simulink model "sgMdl_IO3xx_SPI_Loopback_MasterSyncMultiSlave"  (R2024b)
settings: Solver=FixedStepAuto  StartTime=0.0  StopTime=inf  RelTol=1e-3  EnableMultiTasking=on
undefined symbols (not defined in the file): Pull, pull, up
libraries: simulink x2, speedgoatlib_fpga_spi x2, speedgoatlib_fpga x1
Description:
  | IO3xx SPI - Loopback Master Sync MultiSlave
settings Model: ModifiedByFormat=Speedgoat  SimulationMode=external  ExtModeTrigDuration=100000  Creator=Speedgoat  LastModifiedBy=Speedgoat
settings SolverCC: ConcurrentTasks=on  AlgebraicLoopSolver=TrustRegion  PositivePriorityOrder=on  InsertRTBMode=Never (minimum delay)
settings DataIOCC: SaveFormat=Array  SaveState=on  SignalLoggingName=logsOut
settings OptimizationCC: BlockReduction=off  BooleanDataType=off  OptimizeBlockIOStorage=off  BufferReuse=off  ReuseModelBlockBuffer=off  GlobalBufferReuse=off  ExpressionFolding=off  LocalBlockOutputs=off  InitFltsAndDblsToZero=on  OptimizeDataStoreBuffers=off  BusAssignmentInplaceUpdate=off
settings DebuggingCC: SaveWithParameterizedLinksMsg=none  UnderspecifiedInitializationDetection=Classic  MergeDetectMultiDrivingBlocksExec=none  CheckExecutionContextPreStartOutputMsg=on  SignalResolutionControl=TryResolveAllWithWarning  TasksWithSamePriorityMsg=none  UnconnectedInputMsg=warning  UnconnectedOutputMsg=warning  UnconnectedLineMsg=warning  SFUnexpectedBacktrackingDiag=warning  SFNoUnconditionalDefaultTransitionDiag=warning  SFExecutionAtInitializationDiag=none  ArithmeticOperatorsInVariantConditions=warning
settings HardwareCC: ProdBitPerLong=64  ProdLongLongMode=on  ProdHWDeviceType=Intel->x86-64 (Linux 64)
settings ModelReferenceCC: EnableRefExpFcnMdlSchedulingChecks=on  PropagateSignalLabelsOutOfModel=off
settings SFSimCC: SimUseLocalCustomCode=off  SimTargetLang=C++
settings RTWCC: Description=Speedgoat Real-Time Target Machine  SystemTargetFile=speedgoat.tlc  TemplateMakefile=slrealtime_default_tmf  RTWUseLocalCustomCode=off  Toolchain=Simulink Real-Time Toolchain  BuildConfiguration=Faster Runs  TargetLang=C++  GPUComputeCapability=3.5  DLArmComputeVersion=19.05
settings CodeAppCC: StateflowObjectComments=on
settings SimulinkRealTimeTargetCC: SubcomponentCodeInterfacePackaging=Reusable function  MATLABClassNameForMDSCustomization=Simulink.SoftwareTarget.GRTCustomization  InstructionSetFMA=off  LogToMDFFile=off  SLRTForcePollingMode=on  SLRTFileLogMaxRuns=10  UseGCCFastMath=on
settings ConfigComp: CovMetricSettings=dw  CovSaveCumulativeToWorkspaceVar=on  CovSaveSingleToWorkspaceVar=on  CovExternalEMLEnable=off  CovSFcnEnable=off  CovBoundaryAbsTol=1.0e-5

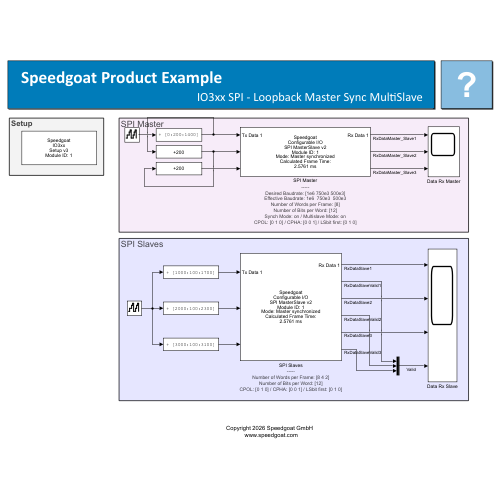
[thumbnail: Simulink's stored preview of the top-level diagram]
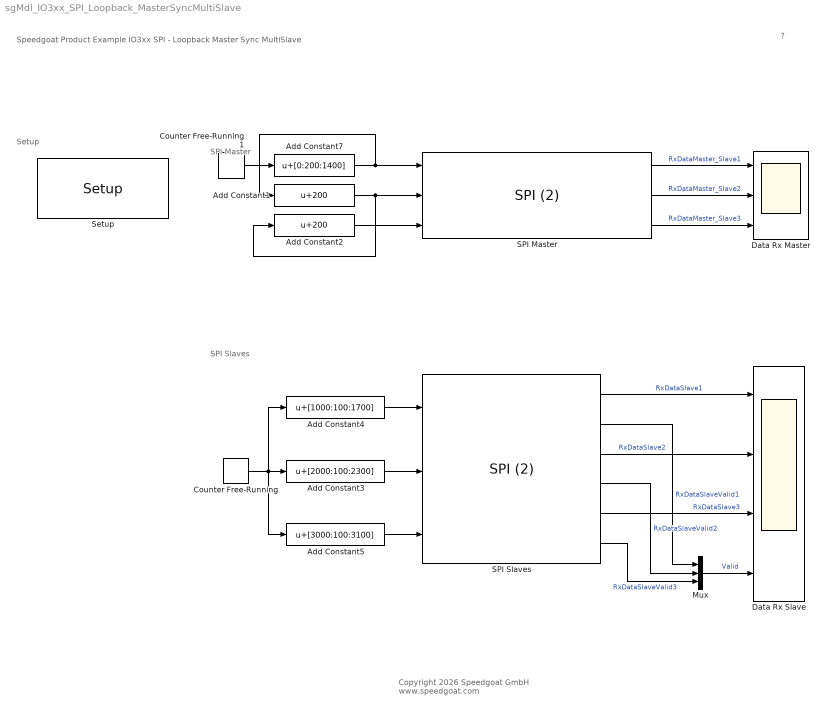
== system sgMdl_IO3xx_SPI_Loopback_MasterSyncMultiSlave ==
  note: SPI Master
  note: Setup
  note: SPI Slaves
  note: Speedgoat Product Example
      | IO3xx SPI - Loopback Master Sync MultiSlave
  note: ?
  note: Copyright 2026 Speedgoat GmbH
      |  www.speedgoat.com
  Add Constant1 : Bias  Bias=200  SaturateOnIntegerOverflow=off
  Add Constant2 : Bias  Bias=200  SaturateOnIntegerOverflow=off
  Add Constant3 : Bias  Bias=[2000:100:2300]  SaturateOnIntegerOverflow=off
  Add Constant4 : Bias  Bias=[1000:100:1700]  SaturateOnIntegerOverflow=off
  Add Constant5 : Bias  Bias=[3000:100:3100]  SaturateOnIntegerOverflow=off
  Add Constant7 : Bias  Bias=[0:200:1400]  SaturateOnIntegerOverflow=off
  Counter Free-Running : simulink/Sources/Counter Free-Running  NumBits=32  tsamp=1e-3
  Counter Free-Running1 : simulink/Sources/Counter Free-Running  NumBits=32  tsamp=1e-3
  Data Rx Master : Scope  NumInputPorts=3
  Data Rx Slave : Scope  NumInputPorts=4
  Mux : Mux  Inputs=3
  SPI Master : speedgoatlib_fpga_spi/SPI (2)  id=1  chan=[1]  samp_time=-1  role=Master  sync_mode=on  multislave_mode=on  write_only=off  read_only=off  multislave_chan=[1 2 3]  cpol=[0 1 0]  cpha=[0 0 1]  frequency=[1e6 750e3 500e3]  frequency_eff="1e6  750e3  500e3"  delay_start=[2e-6]  delay_start_eff=2e-6  delay_interword=[5e-6]  delay_interword_eff=5e-6  delay_stop=[2e-6]  delay_stop_eff=2e-6  delay_compensation=[200e-9]  delay_compensation_eff=200e-9  words_per_frame=[8]  dynamic_words_per_frame=off  bits_per_word=[12]  bit_shift_lsb_first=[0 1 0]  no_cs=off  clock_timeout=[1e-6]  clock_timeout_eff=1E-06  data_sync_length=[5e-6]  data_sync_length_eff=5e-6  data_sync_frame_start=[0]
      settings: SourceProductName=Simulink Real-Time: Speedgoat I/O Blockset
      settings: AttributesFormatString=|
      | -----
      | Desired Baudrate: %<frequency>
      | Effective Baudrate: %<frequency_eff>
      | Number of Words per Frame: %<words_per_frame>
      | Number of Bits per Word: %<bits_per_word>
      | Synch Mode: %<sync_mode> / Multislave Mode: %<multislave_mode>
      | CPOL: %<cpol> / CPHA: %<cpha> / LSbit first: %<bit_shift_lsb_first>
  SPI Slaves : speedgoatlib_fpga_spi/SPI (2)  id=1  chan=[2:4]  samp_time=-1  role=Slave  sync_mode=on  multislave_mode=off  write_only=off  read_only=off  multislave_chan=[1]  cpol=[0 1 0]  cpha=[0 0 1]  frequency=[100e3]  frequency_eff=100e3  delay_start=[100e-9]  delay_start_eff=106.7e-9  delay_interword=[1e-6]  delay_interword_eff=1e-6  delay_stop=[1e-6]  delay_stop_eff=1e-6  delay_compensation=[100e-9]  delay_compensation_eff=106.7e-9  words_per_frame=[8 4 2]  dynamic_words_per_frame=off  bits_per_word=[12]  bit_shift_lsb_first=[0 1 0]  no_cs=off  clock_timeout=[1e-6]  clock_timeout_eff=1E-06  data_sync_length=[5e-6]  data_sync_length_eff=5e-6  data_sync_frame_start=[0]
      settings: SourceProductName=Simulink Real-Time: Speedgoat I/O Blockset
      settings: AttributesFormatString=|
      | -----
      | Number of Words per Frame: %<words_per_frame>
      | Number of Bits per Word: %<bits_per_word>
      | CPOL: %<cpol> / CPHA: %<cpha> / LSbit first: %<bit_shift_lsb_first>
  Setup : speedgoatlib_fpga/Setup/Setup  board=Please select...  id=1  pciSlot=-1  device_id=1  bitstreamFilePath=[]  bitstreamFile=speedgoat_IO306_25k_Comms_test  fpgaFreq=73.73 MHz  enableDma=off  rearEnb_1=off  rearIO_1=None  rearEnb_2=off  rearIO_2=None  ProgSpiFlash=off  ProgBPIFlash=off  useFpgaDmaController=off  dmaTrigDropdown=Model Step  dmaTrigSelect=0  dmaStopOnOverload=on  dmaModeSequential=on  dmaModeParallel=off  PullRPort15=pull-up 3.3V  PullRPort31=pull-up 3.3V  PullRPort47=pull-up 3.3V  PullRPort63=pull-up 3.3V  diffLineTermination_1=on  diffLineTermination_2=on  diffLineTermination_3=on  diffLineTermination_4=on  diffLineTermination_5=on  diffLineTermination_6=on  diffLineTermination_7=on  diffLineTermination_8=on  diffLineTermination_9=on  diffLineTermination_10=on  diffLineTermination_11=on  diffLineTermination_12=on  diffLineTermination_13=on  diffLineTermination_14=on  diffLineTermination_15=on  diffLineTermination_16=on  diffLineTermination_17=on  diffLineTermination_18=on  diffLineTermination_19=on  diffLineTermination_20=on  diffLineTermination_21=on  diffLineTermination_22=on  diffLineTermination_23=on  diffLineTermination_24=on  diffLineTermination_25=on  diffLineTermination_26=on  diffLineTermination_27=on  diffLineTermination_28=on  diffLineTermination_29=on  diffLineTermination_30=on  diffLineTermination_31=on  diffLineTermination_32=on  ioVoltageDropDown1=3.3V  pullResistorDropDown1_1=Pull-up  pullResistorDropDown1_2=Pull-up  pullResistorDropDown1_3=Pull-up  pullResistorDropDown1_4=Pull-up  pullResistorDropDown1_5=Pull-up  pullResistorDropDown1_6=Pull-up  pullResistorDropDown1_7=Pull-up  pullResistorDropDown1_8=Pull-up  ttlIsImplementedCheckBox1=off  pullResistorDropDown2=Pull-up  ioVoltageDropDown2=3.3V  ttlIsImplementedCheckBox2=off  pullResistorDropDown3=Pull-up  ioVoltageDropDown3=3.3V  ttlIsImplementedCheckBox3=off  pullResistorDropDown4=Pull-up  ioVoltageDropDown4=3.3V  ttlIsImplementedCheckBox4=off  pullResistorDropDown5=Pull-up  ioVoltageDropDown5=3.3V  ttlIsImplementedCheckBox5=off  pullResistorDropDown6=Pull-up  ioVoltageDropDown6=3.3V  ttlIsImplementedCheckBox6=off  pullResistorDropDown7=Pull-up  ioVoltageDropDown7=3.3V  ttlIsImplementedCheckBox7=off  pullResistorDropDown8=Pull-up  ioVoltageDropDown8=3.3V  ttlIsImplementedCheckBox8=off  terminationCheckBox1=off  terminationCheckBox2=off  terminationCheckBox3=off  terminationCheckBox4=off  diffIsImplementedCheckBox1=off  terminationCheckBox5=off  terminationCheckBox6=off  terminationCheckBox7=off  terminationCheckBox8=off  diffIsImplementedCheckBox2=off  terminationCheckBox9=off  terminationCheckBox10=off  terminationCheckBox11=off  terminationCheckBox12=off  diffIsImplementedCheckBox3=off  terminationCheckBox13=off  terminationCheckBox14=off  terminationCheckBox15=off  terminationCheckBox16=off  diffIsImplementedCheckBox4=off  terminationCheckBox17=off  terminationCheckBox18=off  terminationCheckBox19=off  terminationCheckBox20=off  diffIsImplementedCheckBox5=off  terminationCheckBox21=off  terminationCheckBox22=off  terminationCheckBox23=off  terminationCheckBox24=off  diffIsImplementedCheckBox6=off  terminationCheckBox25=off  terminationCheckBox26=off  terminationCheckBox27=off  terminationCheckBox28=off  diffIsImplementedCheckBox7=off  terminationCheckBox29=off  terminationCheckBox30=off  terminationCheckBox31=off  terminationCheckBox32=off  diffIsImplementedCheckBox8=off  PullRPort0_1=pull-up  VioPort0_1=3.3V  PullRPort1_1=pull-up  VioPort1_1=3.3V  PullRPort2_1=pull-up  VioPort2_1=3.3V  PullRPort3_1=pull-up  VioPort3_1=3.3V  PullRPort4_1=pull-up  VioPort4_1=3.3V  PullRPort5_1=pull-up  VioPort5_1=3.3V  PullRPort6_1=pull-up  VioPort6_1=3.3V  diffLineTermination_rear1_1=on  diffLineTermination_rear1_2=on  diffLineTermination_rear1_3=on  diffLineTermination_rear1_4=on  diffLineTermination_rear1_5=on  diffLineTermination_rear1_6=on  diffLineTermination_rear1_7=on  diffLineTermination_rear1_8=on  PullRPort0_2=pull-up  VioPort0_2=3.3V  PullRPort1_2=pull-up  VioPort1_2=3.3V  PullRPort2_2=pull-up  VioPort2_2=3.3V  PullRPort3_2=pull-up  VioPort3_2=3.3V  PullRPort4_2=pull-up  VioPort4_2=3.3V  PullRPort5_2=pull-up  VioPort5_2=3.3V  PullRPort6_2=pull-up  VioPort6_2=3.3V  diffLineTermination_rear2_1=on  diffLineTermination_rear2_2=on  diffLineTermination_rear2_3=on  diffLineTermination_rear2_4=on  diffLineTermination_rear2_5=on  diffLineTermination_rear2_6=on  diffLineTermination_rear2_7=on  diffLineTermination_rear2_8=on
      settings: SourceProductName=Simulink Real-Time: Speedgoat I/O Blockset
  wires:
  Counter Free-Running/1 -> Add Constant5/1, Add Constant3/1, Add Constant4/1
  Add Constant4/1 -> SPI Slaves/1
  Counter Free-Running1/1 -> Add Constant7/1
  Add Constant7/1 -> Add Constant1/1, SPI Master/1
  Add Constant2/1 -> SPI Master/3
  SPI Master/1 -> Data Rx Master/1  "RxDataMaster_Slave1"
  SPI Master/2 -> Data Rx Master/2  "RxDataMaster_Slave2"
  SPI Master/3 -> Data Rx Master/3  "RxDataMaster_Slave3"
  Add Constant1/1 -> Add Constant2/1, SPI Master/2
  Add Constant3/1 -> SPI Slaves/2
  Add Constant5/1 -> SPI Slaves/3
  SPI Slaves/1 -> Data Rx Slave/1  "RxDataSlave1"
  SPI Slaves/3 -> Data Rx Slave/2  "RxDataSlave2"
  SPI Slaves/5 -> Data Rx Slave/3  "RxDataSlave3"
  Mux/1 -> Data Rx Slave/4  "Valid"
  SPI Slaves/2 -> Mux/1  "RxDataSlaveValid1"
  SPI Slaves/4 -> Mux/2  "RxDataSlaveValid2"
  SPI Slaves/6 -> Mux/3  "RxDataSlaveValid3"
